simulink model "Regulatoare pentru modelul sursei"  (R2020b)
settings: Solver=VariableStepAuto  StartTime=0.0  StopTime=0.02  RelTol=1e-3
undefined symbols (not defined in the file): C, ku, L, Rs, U21
libraries: simulink x1
settings Model: Creator=tudor  LastModifiedBy=tudor

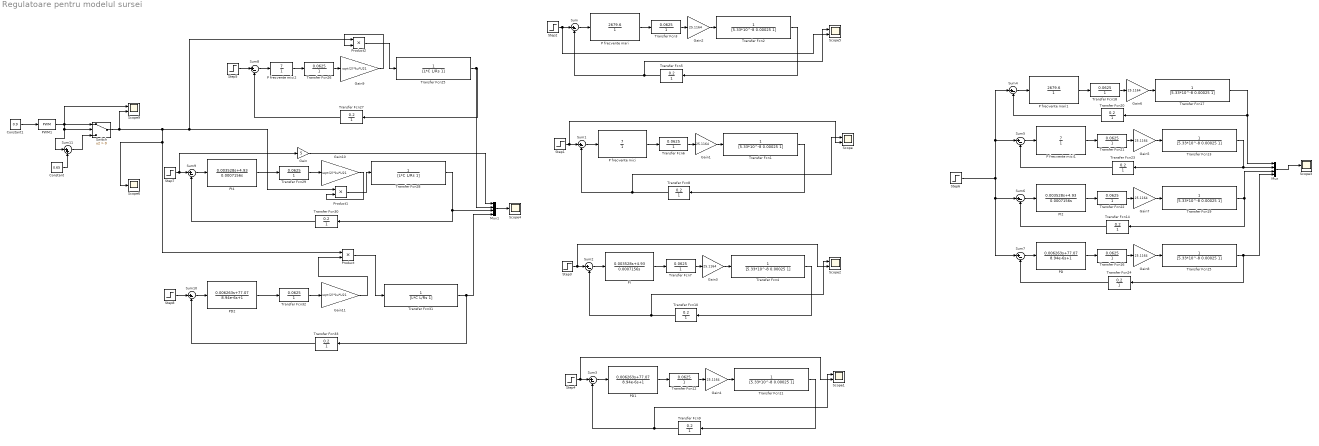
== system Regulatoare pentru modelul sursei ==
  Constant : Constant  Value=0.65
  Constant1 : Constant  Value=0.9  OutMin=[0.65]  OutMax=[1]
  Gain : Gain  Gain=5
  Gain{1..8} (8 alike) : Gain  Gain=25.1164
  Gain10 : Gain  Gain=sqrt(2)*ku*U21
  Gain11 : Gain  Gain=sqrt(2)*ku*U21
  Gain9 : Gain  Gain=sqrt(2)*ku*U21
  Mux : Mux
  Mux1 : Mux
  P frecvente mari : TransferFcn  Numerator=2679.6  Denominator=1
  P frecvente mari1 : TransferFcn  Numerator=2679.6  Denominator=1
  P frecvente mici : TransferFcn  Numerator=7  Denominator=1
  P frecvente mici1 : TransferFcn  Numerator=7  Denominator=1
  P frecvente mici2 : TransferFcn  Numerator=7  Denominator=1
  PD : TransferFcn  Numerator=[0.006263 77.07]  Denominator=[8.94e-6 1]
  PD1 : TransferFcn  Numerator=[0.006263 77.07]  Denominator=[8.94e-6 1]
  PD2 : TransferFcn  Numerator=[0.006263 77.07]  Denominator=[8.94e-6 1]
  PI : TransferFcn  Numerator=[0.003528 4.93]  Denominator=[0.0007156 0]
  PI2 : TransferFcn  Numerator=[0.003528 4.93]  Denominator=[0.0007156 0]
  PI4 : TransferFcn  Numerator=[0.003528 4.93]  Denominator=[0.0007156 0]
  PWM1 : simulink/Discontinuities/PWM  DisableCoverage=on  Period=0.02/2.7  DisallowZeroDutyCycle=off  RunAtFixedTimeIntervals=off  SampleTime=0.1
  Product : Product
  Product1 : Product
  Product2 : Product
  Scope{,1..2,5,9} (5 alike) : Scope  NumInputPorts=2
  Scope3 : Scope
  Scope4 : Scope
  Scope6 : Scope
  Step{1..8} (8 alike) : Step  Time=0.0001  After=2.5  SampleTime=0
  Sum{,1..10} (11 alike) : Sum  Inputs=|+-
  Sum11 : Sum  Inputs=|++
  Switch : Switch  Criteria=u2 > Threshold
  Transfer Fcn{1..2,4,11,13,15,17,19} (8 alike) : TransferFcn  Numerator=1  Denominator=[5.33*10^-8 0.00025 1]
  Transfer Fcn{5,8..10,14,20,23..24,27,30,33} (11 alike) : TransferFcn  Numerator=0.2  Denominator=1
  Transfer Fcn{3,6..7,12,16,18,21..22,26,29,32} (11 alike) : TransferFcn  Numerator=[0.0625]  Denominator=1
  Transfer Fcn25 : TransferFcn  Numerator=1  Denominator=[L*C L/Rs 1]
  Transfer Fcn28 : TransferFcn  Numerator=1  Denominator=[L*C L/Rs 1]
  Transfer Fcn31 : TransferFcn  Numerator=1  Denominator=[L*C L/Rs 1]
  wires:
  Sum/1 -> P frecvente mari/1
  Gain2/1 -> Transfer Fcn2/1
  Step2/1 -> Scope5/2, Sum/1
  Transfer Fcn3/1 -> Gain2/1
  Transfer Fcn2/1 -> Transfer Fcn5/1
  Transfer Fcn5/1 -> Scope5/1, Sum/2
  P frecvente mari/1 -> Transfer Fcn3/1
  Gain1/1 -> Transfer Fcn1/1
  Transfer Fcn1/1 -> Transfer Fcn8/1
  Sum1/1 -> P frecvente mici/1
  Step1/1 -> Scope/2, Sum1/1
  P frecvente mici/1 -> Transfer Fcn6/1
  Transfer Fcn8/1 -> Scope/1, Sum1/2
  Transfer Fcn6/1 -> Gain1/1
  Gain3/1 -> Transfer Fcn4/1
  Transfer Fcn4/1 -> Transfer Fcn10/1
  Sum2/1 -> PI/1
  Step3/1 -> Scope2/2, Sum2/1
  PI/1 -> Transfer Fcn7/1
  Transfer Fcn10/1 -> Scope2/1, Sum2/2
  Transfer Fcn7/1 -> Gain3/1
  Sum3/1 -> PD1/1
  PD1/1 -> Transfer Fcn12/1
  Transfer Fcn11/1 -> Transfer Fcn9/1
  Transfer Fcn9/1 -> Scope1/1, Sum3/2
  Transfer Fcn12/1 -> Gain4/1
  Step4/1 -> Scope1/2, Sum3/1
  Gain4/1 -> Transfer Fcn11/1
  Transfer Fcn15/1 -> Mux/4, Transfer Fcn24/1
  Transfer Fcn16/1 -> Gain8/1
  Gain8/1 -> Transfer Fcn15/1
  Transfer Fcn17/1 -> Mux/1, Transfer Fcn20/1
  Transfer Fcn20/1 -> Sum4/2
  Transfer Fcn24/1 -> Sum7/2
  Transfer Fcn22/1 -> Gain7/1
  PD/1 -> Transfer Fcn16/1
  Sum7/1 -> PD/1
  P frecvente mari1/1 -> Transfer Fcn18/1
  Sum4/1 -> P frecvente mari1/1
  Transfer Fcn14/1 -> Sum6/2
  Transfer Fcn19/1 -> Transfer Fcn14/1, Mux/3
  Sum6/1 -> PI2/1
  Transfer Fcn23/1 -> Sum5/2
  P frecvente mici1/1 -> Transfer Fcn21/1
  PI2/1 -> Transfer Fcn22/1
  Transfer Fcn21/1 -> Gain5/1
  Gain7/1 -> Transfer Fcn19/1
  Sum5/1 -> P frecvente mici1/1
  Gain5/1 -> Transfer Fcn13/1
  Transfer Fcn13/1 -> Mux/2, Transfer Fcn23/1
  Transfer Fcn18/1 -> Gain6/1
  Gain6/1 -> Transfer Fcn17/1
  Step6/1 -> Sum7/1, Sum6/1, Sum4/1, Sum5/1
  Mux/1 -> Scope3/1
  Transfer Fcn25/1 -> Mux1/2, Transfer Fcn27/1
  Gain9/1 -> Product2/2
  Step5/1 -> Sum8/1
  Transfer Fcn27/1 -> Sum8/2
  P frecvente mici2/1 -> Transfer Fcn26/1
  Transfer Fcn26/1 -> Gain9/1
  Sum8/1 -> P frecvente mici2/1
  PI4/1 -> Transfer Fcn29/1
  Sum9/1 -> PI4/1
  Transfer Fcn29/1 -> Gain10/1
  Transfer Fcn30/1 -> Sum9/2
  Gain10/1 -> Product1/2
  Transfer Fcn28/1 -> Mux1/3, Transfer Fcn30/1
  Step7/1 -> Gain/1, Sum9/1
  PD2/1 -> Transfer Fcn32/1
  Sum10/1 -> PD2/1
  Transfer Fcn32/1 -> Gain11/1
  Transfer Fcn33/1 -> Sum10/2
  Transfer Fcn31/1 -> Transfer Fcn33/1, Mux1/4
  Step8/1 -> Sum10/1
  Gain/1 -> Mux1/1
  Mux1/1 -> Scope4/1
  Switch/1 -> Product2/1, Product1/1, Scope6/1, Product/1, Scope9/2
  Gain11/1 -> Product/2
  Product/1 -> Transfer Fcn31/1
  Product1/1 -> Transfer Fcn28/1
  Product2/1 -> Transfer Fcn25/1
  PWM1/1 -> Sum11/1, Switch/2, Switch/1, Scope9/1
  Constant1/1 -> PWM1/1
  Constant/1 -> Sum11/2
  Sum11/1 -> Switch/3
